simulink model "BMS_SOC_2023"  (R2023b)
settings: Solver=ode4  StartTime=0.0  StopTime=durata_totale  FixedStep=0.1  MaxStep=1  RelTol=1e-3
undefined symbols (not defined in the file or in its folder): batt, cell, metadata, pack
libraries: simulink x3
settings Model: SimulationMode=accelerator  Creator=39327  LastModifiedBy=faxio
settings DebuggingCC: UnconnectedInputMsg=warning  UnconnectedOutputMsg=warning  UnconnectedLineMsg=warning
settings ModelReferenceCC: EnableRefExpFcnMdlSchedulingChecks=on
settings RTWCC: DLArmComputeVersion=19.05
settings ConfigComp: CovBoundaryAbsTol=1.0e-5

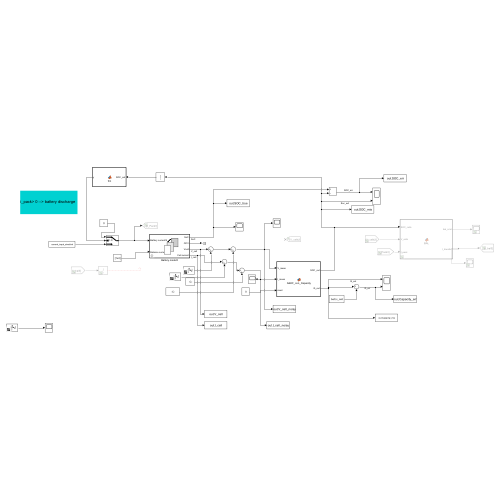
[thumbnail: Simulink's stored preview of the top-level diagram]
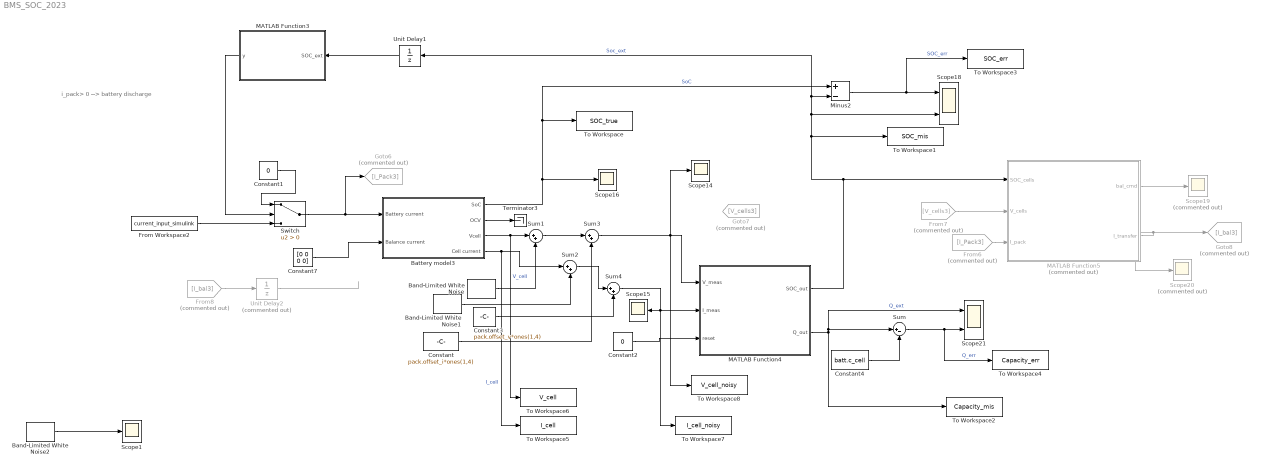
== system BMS_SOC_2023 ==
  note: i_pack> 0 --> battery discharge
  Band-Limited White Noise : simulink/Sources/Band-Limited White Noise  Cov=[pack.sigma_v]  Ts=0.1  seed=[23341]
  Band-Limited White Noise1 : simulink/Sources/Band-Limited White Noise  Cov=[pack.sigma_i]  Ts=0.1  seed=[23341]
  Band-Limited White Noise2 : simulink/Sources/Band-Limited White Noise  Cov=0.0000001  Ts=0.1  seed=[23341]
  Battery model3 : Subsystem  mask{Soc_init=batt.soc0*0.9, Qcell=batt.c_cell, R0_data=batt.r0, R1=batt.r1, C1=batt.c1, ocv_data=cell.ocv, soc_data=cell.soc}
      mask prompts: Soc_init "initial SoC [N_cell*1]"; Qcell "cell capacity [N_cell*1]"; R0_data "R0 [Ncell*soc_pnt]"; R1 "R1[not used here]"; C1 "C1[not used here]"; ocv_data "ocv_data [1*soc_pnt]"; soc_data "soc_data [1*soc_pnt]"
      mask DialogControl DescGroupVar Prompt: Battery model composed of Ncell
      mask DialogControl DescTextVar Prompt: the SoC varies in range 0-1.  Cell number is defined with the dimension of "cell capacity"[N_cell]
  Constant : Constant  Value=pack.offset_i*ones(1,4)
  Constant1 : Constant  Value=0
  Constant2 : Constant  Value=0
  Constant3 : Constant  Value=pack.offset_v*ones(1,4)
  Constant4 : Constant  Value=batt.c_cell
  Constant7 : Constant  Value=[0 0 0 0]
  From Workspace2 : FromWorkspace  VariableName=current_input_simulink  SampleTime=1
  From6 : From  Commented=on  GotoTag=I_Pack3
  From7 : From  Commented=on  GotoTag=V_cells3
  From8 : From  Commented=on  GotoTag=I_bal3
  Goto6 : Goto  Commented=on  GotoTag=I_Pack3
  Goto7 : Goto  Commented=on  GotoTag=V_cells3
  Goto8 : Goto  Commented=on  GotoTag=I_bal3
  MATLAB Function3 : MATLAB Function  TreatAsAtomicUnit=on
  MATLAB Function4 : MATLAB Function  TreatAsAtomicUnit=on
  MATLAB Function5 : MATLAB Function  Commented=on  TreatAsAtomicUnit=on  SystemSampleTime=0.1
  Minus2 : Sum  Inputs=+-
  Scope{1,14..16} (4 alike) : Scope
  Scope18 : Scope  NumInputPorts=2
  Scope19 : Scope  Commented=on
  Scope20 : Scope  Commented=on
  Scope21 : Scope  NumInputPorts=2
  Sum : Sum  Inputs=|+-
  Sum{1..4} (4 alike) : Sum  Inputs=|++
  Switch : Switch  Criteria=u2 > Threshold  SaturateOnIntegerOverflow=off  InputSameDT=off
  Terminator3 : Terminator
  To Workspace : ToWorkspace  VariableName=SOC_true  SaveFormat=Timeseries  SampleTime=-1
  To Workspace1 : ToWorkspace  VariableName=SOC_mis  SaveFormat=Timeseries  SampleTime=-1
  To Workspace2 : ToWorkspace  VariableName=Capacity_mis  SaveFormat=Timeseries  SampleTime=-1
  To Workspace3 : ToWorkspace  VariableName=SOC_err  SaveFormat=Timeseries  SampleTime=-1
  To Workspace4 : ToWorkspace  VariableName=Capacity_err  SaveFormat=Timeseries  SampleTime=-1
  To Workspace5 : ToWorkspace  VariableName=I_cell  SaveFormat=Timeseries  SampleTime=-1
  To Workspace6 : ToWorkspace  VariableName=V_cell  SaveFormat=Timeseries  SampleTime=-1
  To Workspace7 : ToWorkspace  VariableName=I_cell_noisy  SaveFormat=Timeseries  SampleTime=-1
  To Workspace8 : ToWorkspace  VariableName=V_cell_noisy  SaveFormat=Timeseries  SampleTime=-1
  Unit Delay1 : UnitDelay  SampleTime=-1  HasFrameUpgradeWarning=on
  Unit Delay2 : UnitDelay  Commented=on  SampleTime=-1  HasFrameUpgradeWarning=on
  wires:
  MATLAB Function5/2(I_transfer) -> Scope20/1, Goto8/1
  Battery model3/3(Vcell) -> Sum1/1, To Workspace6/1  "V_cell"
  From8/1 -> Unit Delay2/1
  Unit Delay2/1 -> ?
  Battery model3/4(Cell current) -> To Workspace5/1, Sum2/1  "I_cell"
  From7/1 -> MATLAB Function5/2(V_cells)
  From6/1 -> MATLAB Function5/3(I_pack)
  MATLAB Function5/1(bal_cmd) -> Scope19/1
  Battery model3/1(SoC) -> Minus2/1, To Workspace/1, Scope16/1  "SoC"
  Minus2/1 -> To Workspace3/1, Scope18/1  "SOC_err"
  Battery model3/2(OCV) -> Terminator3/1
  MATLAB Function4/2(Q_out) -> Scope21/1, Sum/1, To Workspace2/1  "Q_ext"
  Constant2/1 -> MATLAB Function4/3(reset)
  Constant4/1 -> Sum/2
  Sum/1 -> To Workspace4/1, Scope21/2  "Q_err"
  MATLAB Function4/1(SOC_out) -> Scope18/2, Unit Delay1/1, Minus2/2, To Workspace1/1, MATLAB Function5/1(SOC_cells)  "Soc_ext"
  Constant7/1 -> Battery model3/2(Balance current)
  From Workspace2/1 -> Switch/3
  Switch/1 -> Goto6/1, Battery model3/1(Battery current)
  MATLAB Function3/1(y) -> Switch/2
  Unit Delay1/1 -> MATLAB Function3/1(SOC_ext)
  Constant1/1 -> Switch/1
  Sum1/1 -> Sum3/1
  Band-Limited White Noise/1 -> Sum1/2
  Band-Limited White Noise1/1 -> Sum2/2
  Sum3/1 -> Scope14/1, To Workspace8/1, MATLAB Function4/1(V_meas)
  Sum2/1 -> Sum4/1
  Sum4/1 -> MATLAB Function4/2(I_meas), To Workspace7/1, Scope15/1
  Constant/1 -> Sum3/2
  Constant3/1 -> Sum4/2
  Band-Limited White Noise2/1 -> Scope1/1

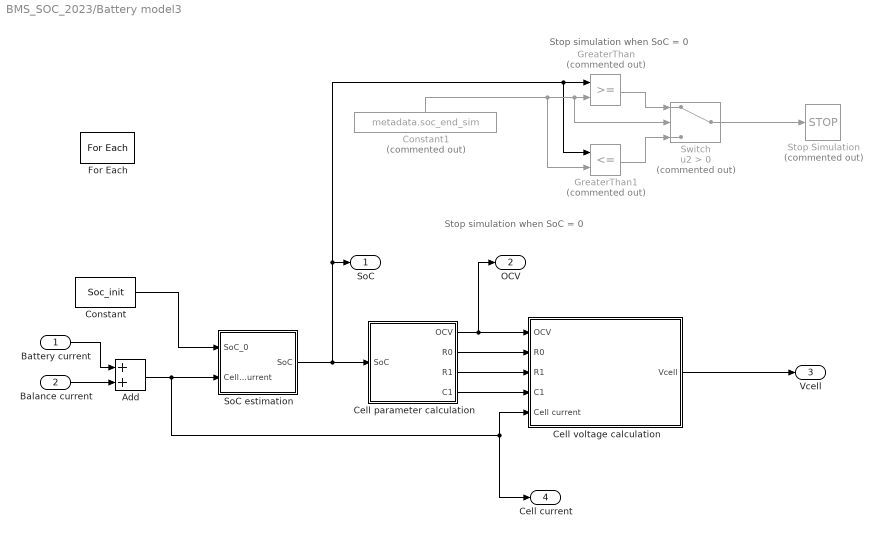
== system BMS_SOC_2023/Battery model3 ==
  note: Stop simulation when SoC = 0
  note: Stop simulation when SoC = 0
  Battery current : Inport
  Balance current : Inport  Port=2  Partition=on  PartitionDimension=1  PartitionWidth=1  PartitionOffset=0
  Add : Sum
  Cell parameter calculation : Subsystem
  Cell voltage calculation : Subsystem
  Constant : Constant  Value=Soc_init
  Constant1 : Constant  Commented=on  Value=metadata.soc_end_sim
  For Each : ForEach  DisableCoverage=on  IterateSubsysMaskParameter=on,on,on,off,off,off,off
  GreaterThan : RelationalOperator  Commented=on  OutDataTypeStr=boolean  RndMeth=Simplest  InputSameDT=off
  GreaterThan1 : RelationalOperator  Commented=on  Operator=<=  OutDataTypeStr=boolean  RndMeth=Simplest  InputSameDT=off
  SoC estimation : Subsystem
  Stop Simulation : Stop  Commented=on
  Switch : Switch  Commented=on  Criteria=u2 > Threshold  SaturateOnIntegerOverflow=off  InputSameDT=off
  SoC : Outport  ConcatenationDimension=1
  OCV : Outport  Port=2  ConcatenationDimension=1
  Vcell : Outport  Port=3  ConcatenationDimension=1
  Cell current : Outport  Port=4  ConcatenationDimension=1
  wires:
  Add/1 -> Cell voltage calculation/5(Cell current), Cell current/1, SoC estimation/2(Cell current)
  Constant/1 -> SoC estimation/1(SoC_0)
  SoC estimation/1(SoC) -> GreaterThan/1, GreaterThan1/1, SoC/1, Cell parameter calculation/1(SoC)
  Cell parameter calculation/4(C1) -> Cell voltage calculation/4(C1)
  Cell parameter calculation/3(R1) -> Cell voltage calculation/3(R1)
  Cell parameter calculation/2(R0) -> Cell voltage calculation/2(R0)
  Cell parameter calculation/1(OCV) -> OCV/1, Cell voltage calculation/1(OCV)
  Cell voltage calculation/1(Vcell) -> Vcell/1
  Battery current/1 -> Add/1
  Balance current/1 -> Add/2
  Constant1/1 -> GreaterThan/2, Switch/2, GreaterThan1/2
  Switch/1 -> Stop Simulation/1
  GreaterThan/1 -> Switch/1
  GreaterThan1/1 -> Switch/3

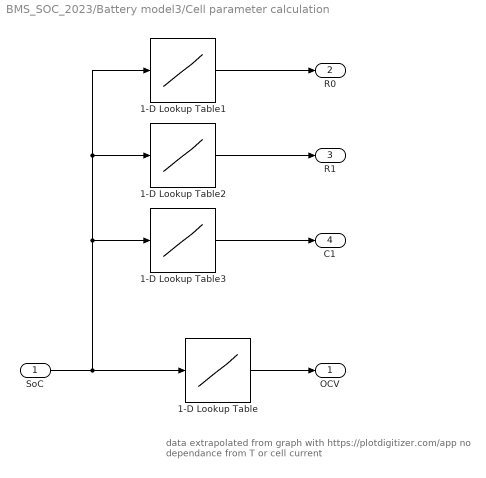
== system BMS_SOC_2023/Battery model3/Cell parameter calculation ==
  note: data extrapolated from graph with https://plotdigitizer.com/app
      |
      | no dependance from T or cell current
  SoC : Inport
  1-D Lookup Table : Lookup_n-D  NumberOfTableDimensions=1  BreakpointsForDimension1=cell.soc  Table=cell.ocv  InternalRulePriority=Speed  RndMeth=Simplest
  1-D Lookup Table1 : Lookup_n-D  NumberOfTableDimensions=1  BreakpointsForDimension1=cell.soc  Table=cell.r0  InternalRulePriority=Speed  RndMeth=Simplest
  1-D Lookup Table2 : Lookup_n-D  NumberOfTableDimensions=1  BreakpointsForDimension1=cell.soc  Table=cell.r1  InternalRulePriority=Speed  RndMeth=Simplest
  1-D Lookup Table3 : Lookup_n-D  NumberOfTableDimensions=1  BreakpointsForDimension1=cell.soc  Table=cell.c1  InternalRulePriority=Speed  RndMeth=Simplest
  OCV : Outport
  R0 : Outport  Port=2
  R1 : Outport  Port=3
  C1 : Outport  Port=4
  wires:
  1-D Lookup Table/1 -> OCV/1
  SoC/1 -> 1-D Lookup Table3/1, 1-D Lookup Table2/1, 1-D Lookup Table1/1, 1-D Lookup Table/1
  1-D Lookup Table1/1 -> R0/1
  1-D Lookup Table3/1 -> C1/1
  1-D Lookup Table2/1 -> R1/1

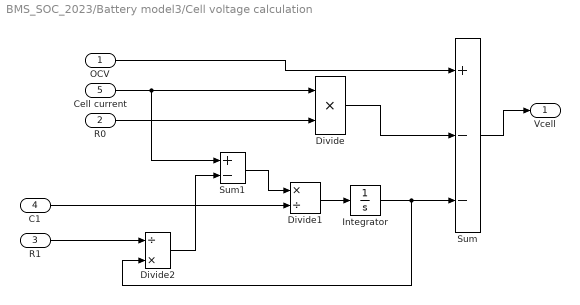
== system BMS_SOC_2023/Battery model3/Cell voltage calculation ==
  OCV : Inport
  R0 : Inport  Port=2
  R1 : Inport  Port=3
  C1 : Inport  Port=4
  Cell current : Inport  Port=5
  Divide : Product  Inputs=**
  Divide1 : Product  Inputs=*/
  Divide2 : Product  Inputs=/*
  Integrator : Integrator
  Sum : Sum  Inputs=+--
  Sum1 : Sum  Inputs=+-
  Vcell : Outport
  wires:
  Sum/1 -> Vcell/1
  OCV/1 -> Sum/1
  Divide/1 -> Sum/2
  Cell current/1 -> Sum1/1, Divide/1
  R0/1 -> Divide/2
  Divide1/1 -> Integrator/1
  Integrator/1 -> Sum/3, Divide2/2
  Sum1/1 -> Divide1/1
  Divide2/1 -> Sum1/2
  C1/1 -> Divide1/2
  R1/1 -> Divide2/1

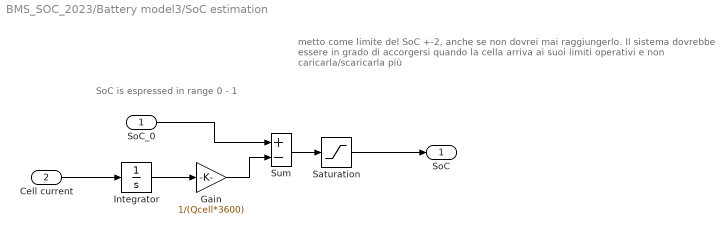
== system BMS_SOC_2023/Battery model3/SoC estimation ==
  note: metto come limite del SoC +-2, anche se non dovrei mai raggiungerlo. Il sistema dovrebbe essere in grado di accorgersi quando la cella arriva ai suoi limiti operativi e non caricarla/scaricarla più
  note: SoC is espressed in range 0 - 1
  SoC_0 : Inport
  Cell current : Inport  Port=2
  Gain : Gain  Gain=1/(Qcell*3600)
  Integrator : Integrator
  Saturation : Saturate  UpperLimit=2  LowerLimit=-2
  Sum : Sum  Inputs=+-
  SoC : Outport
  wires:
  Saturation/1 -> SoC/1
  Integrator/1 -> Gain/1
  Cell current/1 -> Integrator/1
  Sum/1 -> Saturation/1
  Gain/1 -> Sum/2
  SoC_0/1 -> Sum/1

== matlab function BMS_SOC_2023/MATLAB Function3 ==
  data: SOC_ext input; y output
function y = fcn(SOC_ext)

y = any(SOC_ext<0.1)||any(SOC_ext>0.95);

== matlab function BMS_SOC_2023/MATLAB Function4 ==
  settings: updateMethod=DISCRETE  sampleTime=0.1
  data: SOC_out output; Q_out output; V_meas input; I_meas input; reset input; batt_param parameter
function [SOC_out, Q_out]  = AEKF_con_Capacity(V_meas, I_meas, reset,batt_param)  %#codegen

% Ingressi:
%   V_meas - Vettore tensioni misurate [n_cells x 1]
%   I_meas - Vettore correnti misurate [n_cells x 1]  
%   reset  - Segnale di reset (booleano)
%
% Uscita:
%   SOC_out - SOC stimato [n_cells x 1]
%   Q_out   - Capacità stimata [n_cells x 1]


    M=10; %finestra di misura per AEKF
    % Numero di celle 
    n_cells = 4;

    % Parametri batteria
    Ts = 0.1;           % Tempo campionamento [s]
    Q_cell = batt_param.c_cell;        % Capacità nominale [Ah]
    R0_matrix = batt_param.r0;         % Resistenza ohmica [Ohm]
    R1_matrix = batt_param.r1;         % Resistenza RC [Ohm]
    C1_matrix = batt_param.c1;          % Capacità RC [F]
    
    SOC_grid =batt_param.soc(:);
    OCV_tab  =batt_param.ocv(:);




    % Pre-calcola derivata OCV
    n_points = length(SOC_grid);
    dSOC = SOC_grid(2) - SOC_grid(1);
    dOCV_temp = diff(OCV_tab) / dSOC;
    dOCV_tab = zeros(n_points, 1);
    dOCV_tab(1) = dOCV_temp(1);
    for i = 2:n_points-1
        dOCV_tab(i) = dOCV_temp(i);
    end
    dOCV_tab(n_points) = dOCV_temp(n_points-1);
     
    % % Rumore EKF
    % Q_cov = diag([1e-5, 1e-3, 1e-8]);
    % R_var = 0.00001;
    
   persistent SOC_state V1_state Q_state P_state H_k_vector Q_cov R_var initialized

if isempty(initialized) || reset
    SOC_state = 0.5 * ones(n_cells,1);
    V1_state  = zeros(n_cells,1);
    Q_state   = Q_cell(:); % inizializza con capacità nominale
    P_state   = zeros(3,3,n_cells);
    
    H_k_vector=    zeros(1,M);
    Q_cov = diag([1e-5, 1e-3, 1e-10]); % rumore piccolo inizialmente su Q (variazione lenta)
    R_var = 0.00001;
    
    for k = 1:n_cells
        P_state(:,:,k) = diag([0.05, 0.01, 1e-3]);
    end
    initialized = true;
end

%% PRE-ALLOCAZIONE

SOC_out = zeros(n_cells,1);
Q_out   = zeros(n_cells,1);
    H_k=0;
%% EKF PER OGNI CELLA

for k = 1:n_cells

    % Stato corrente
    x = [SOC_state(k); V1_state(k); Q_state(k)];
    P = P_state(:,:,k);

    I_k = I_meas(k);
    V_k = V_meas(k);

    %% PREDIZIONE 
    % Coulomb counting
    Q_k = max(1e-6, x(3)); % fa evitare divisione per zero
    SOC_pred = x(1) - (Ts * I_k) / (Q_k * 3600);
    SOC_pred = max(0, min(1, SOC_pred)); %limito il soc tra 0 e 1
    
    % ESTRAGGO LA RIGA k DALLA MATRICE E FACCIO L'INTERPOLAZIONE
    R0_row = R0_matrix(k, :);  % Riga k, vettore [1 x 21]
    R1_row = R1_matrix(k, :);  % Riga k, vettore [1 x 21]
    C1_row = C1_matrix(k, :);  % Riga k, vettore [1 x 21]
        
    % Converte a colonna per interp1
    R0_col = R0_row(:);  % [21 x 1]
    R1_col = R1_row(:);  % [21 x 1]
    C1_col = C1_row(:);  % [21 x 1]

    % Interpolazione
    R0 = interp1(SOC_grid, R0_col, SOC_pred, 'linear', 'extrap');
    R1 = interp1(SOC_grid, R1_col, SOC_pred, 'linear', 'extrap');
    C1 = interp1(SOC_grid, C1_col, SOC_pred, 'linear', 'extrap');
    
    R0=R0*Q_k/Q_cell(k);
    R1=R1*Q_k/Q_cell(k);
    C1=C1*Q_k/Q_cell(k);

    tau1  = R1 * C1;
    alpha = exp(-Ts / tau1);

    % Dinamica RC
    V1_pred = alpha * x(2) + R1 * (1 - alpha) * I_k;

    % Q pred
    Q_pred = x(3);

    x_pred = [SOC_pred; V1_pred; Q_pred];

    % Jacobiano stato
    dSOCdQ = (Ts * I_k) / (Q_k^2 * 3600);
    A = [1, 0, dSOCdQ;
         0, alpha, 0;
         0, 0, 1];

    P_pred = A * P * A' + Q_cov;

    %% AGGIORNAMENTO
    OCV  = interp1(SOC_grid, OCV_tab, SOC_pred,"linear","extrap");
    dOCV = interp1(SOC_grid, dOCV_tab, SOC_pred,"linear","extrap");
        
    V_pred = OCV - x_pred(2) - R0 * I_k;
    y_tilde = V_k - V_pred;

    C_mat = [dOCV, -1, 0];

    S = C_mat * P_pred * C_mat' + R_var;
    K = (P_pred * C_mat') / S;

    % Aggiornamento stato
    x_upd = x_pred + K * y_tilde;
    x_upd(1) = max(0, min(1, x_upd(1)));
    x_upd(3) = max(1e-6, x_upd(3)); % capacità sempre positiva

    % Aggiornamento covarianza
    I3 = eye(3);
    P_upd = (I3 - K * C_mat) * P_pred;

    H_k_vector=circshift(H_k_vector,1);
    H_k_vector(1)=y_tilde*y_tilde';
    if H_k_vector(M)~=0
        H_k=sum(H_k_vector)/M;
        Q_cov=K*H_k*K';
        R_var=H_k-C_mat*P_upd*C_mat';
    end

    Qmin = 0.4 * Q_cell(k);
    Qmax = 1.1 * Q_cell(k);
    x_upd(3) = min(Qmax, max(Qmin, x_upd(3)));

    %% SALVATAGGIO 
    SOC_state(k) = x_upd(1);
    V1_state(k)  = x_upd(2);
    Q_state(k)   = x_upd(3);
    P_state(:,:,k) = P_upd;
    
    
    SOC_out(k) = x_upd(1);
    Q_out(k)   = x_upd(3);
   

end
end

== matlab function BMS_SOC_2023/MATLAB Function5 ==
  settings: updateMethod=DISCRETE  sampleTime=0.1
  data: SOC_cells input; bal_cmd output; V_cells input; I_pack input; I_transfer output; batt_param parameter
function [bal_cmd, I_transfer] = BAL(SOC_cells, V_cells, I_pack, batt_param)

    n_cells = 4;
    
    I_bal_max = batt_param.I_bal_max;
    eta_dcdc = batt_param.eta_dcdc;
    SOC_threshold = batt_param.SOC_threshold;
    V_min_bal = batt_param.V_min_bal;
    V_max_bal = batt_param.V_max_bal;
    
    bal_cmd = zeros(4, 1);
    I_transfer = zeros(4, 1);
    
    % Trova SOC max e min
    SOC_min = SOC_cells(1);
    SOC_max = SOC_cells(1);
    idx_min = 1;
    idx_max = 1;
    
    for k = 1:n_cells
        if SOC_cells(k) < SOC_min
            SOC_min = SOC_cells(k);
            idx_min = k;
        end
        if SOC_cells(k) > SOC_max
            SOC_max = SOC_cells(k);
            idx_max = k;
        end
    end
    
    SOC_range = SOC_max - SOC_min;
    
    % Bilancia se necessario
    if SOC_range > SOC_threshold
        
        V_source = V_cells(idx_max);
        V_dest = V_cells(idx_min);
        
        safe = (V_source > V_min_bal) && (V_source < V_max_bal) && ... 
               (V_dest > V_min_bal) && (V_dest < V_max_bal);
        
        if safe
            I_bal = min(5 * SOC_range * I_bal_max, I_bal_max);
            
            bal_cmd(idx_max) = 1;
            I_transfer(idx_max) = I_bal;
            
            bal_cmd(idx_min) = -1;
            I_transfer(idx_min) = -I_bal * eta_dcdc;
        end
    end
    
end
